simulink model "nonlinearzsystemController1"  (R2020b)
settings: Solver=VariableStepAuto  StartTime=0.0  StopTime=10.0  RelTol=1e-3
settings Model: Creator=Javad  LastModifiedBy=Javad
settings SolverCC: ZeroCrossAlgorithm=Adaptive
settings DebuggingCC: IgnoredZcDiagnostic=none

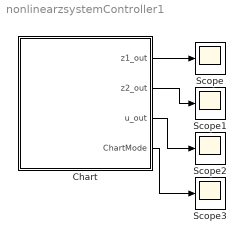
== system nonlinearzsystemController1 ==
  Chart : Stateflow chart  TreatAsAtomicUnit=on
  Scope{,1..3} (4 alike) : Scope
  wires:
  Chart/3(u_out) -> Scope2/1
  Chart/2(z2_out) -> Scope1/1
  Chart/1(z1_out) -> Scope/1
  Chart/4(ChartMode) -> Scope3/1

== stateflow chart nonlinearzsystemController1/Chart ==
  settings: updateMethod=CONTINUOUS
  state Q2
    du:
    z1_dot=-30*z1-20*z2-30*x1_eq-20*x2_eq+24+20*(1.432*z1+0.372*z2);
    z2_dot=0.05*z1+0.1*z2+0.05*x1_eq-0.07;
    z1_out=z1;
    z2_out=z2;
    u_out=1.432*z1+0.372*z2;
  state Q1
    du:
    z1_dot=-30*z1 - 20*z2 - 30*x1_eq - 20*x2_eq + 24 + 20*(1.39*z1-0.329*z2);
    z2_dot=0.05*z1-0.25*z2+0.05*x1_eq-0.25*x2_eq;
    z1_out=z1;
    z2_out=z2;
    u_out=1.39*z1-0.329*z2;
  state Q3
    du:
    z1_dot=-30*z1-20*z2+24-30*x1_eq-20*x2_eq+20*(1.379*z1-0.484*z2);
    z2_dot=0.05*z1-0.2*z2+0.05*x1_eq+0.11;
    z1_out=z1;
    z2_out=z2;
    u_out=1.379*z1-0.484*z2;
  (default) -> Q1 : {z1=0.5-x1_eq;
      | z2=0.1-x2_eq;}
  Q2 -> Q1 [order 2] : [z2<0.2-x2_eq]
  Q1 -> Q2 : [z2>=0.2-x2_eq]
  Q2 -> Q3 [order 1] : [z2>=0.6-x2_eq]
  Q3 -> Q2 : [z2<0.6-x2_eq]
  data: z1_out output; z2_out output; u_out output; z2 local; z1 local; x1_eq constant double =0.3714; x2_eq constant double =0.6429; ChartMode output Enum: ChartModeType
  data z2 settings: updateMethod=SF_CONTINUOUS_TIME_DATA
  data z1 settings: updateMethod=SF_CONTINUOUS_TIME_DATA
